simulink model "Therealone"  (R2023b)
settings: Solver=VariableStepAuto  StartTime=0.0  StopTime=1  RelTol=1e-3
libraries: spsSeriesRLCBranchLib x4, spsDiodeLib x3, spsMeanLib x2, spsCurrentMeasurementLib x2, spsPVArrayLib x2, spsVoltageMeasurementLib x2, spsIGBTDiodeLib x1, sps_lib x1
settings Model: Creator=PC  LastModifiedBy=PC
settings DataIOCC: ReturnWorkspaceOutputs=off

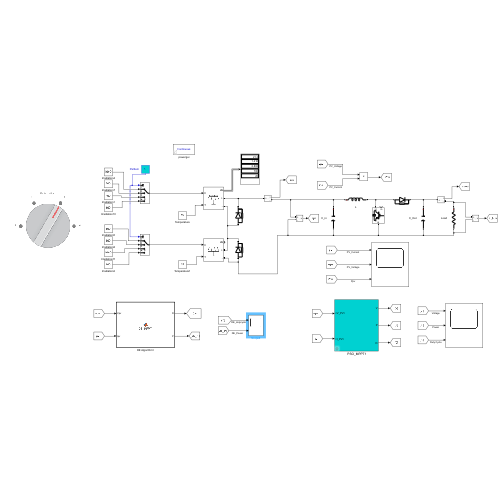
[thumbnail: Simulink's stored preview of the top-level diagram]
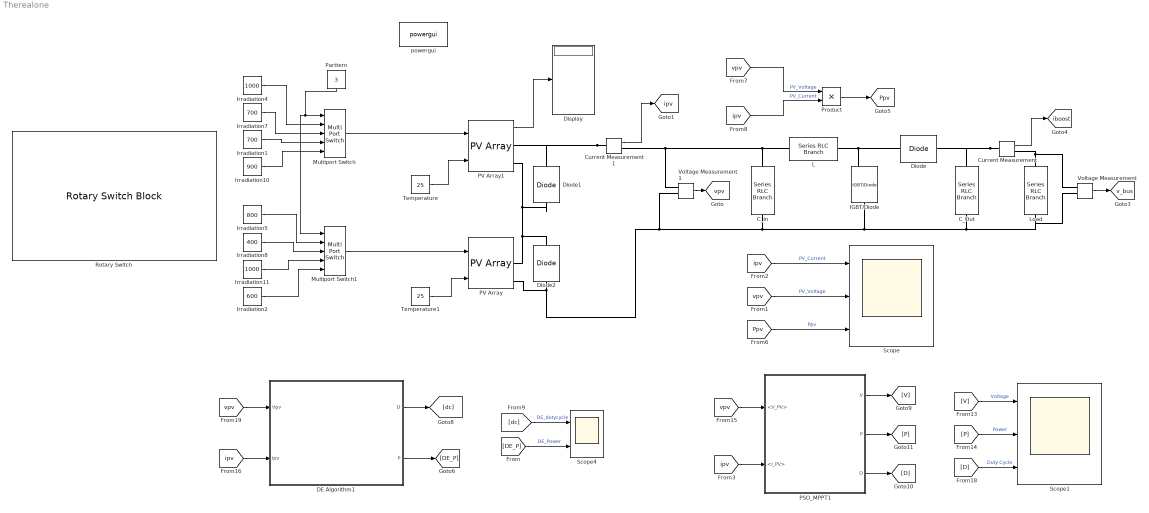
== system Therealone ==
  " PSO_MPPT1" : Subsystem  mask(MPPT PSO Block){Fsw=7812.5, n=4, w=0.1, c1=1, c2=1}
      mask prompts: Fsw "PWM Switching frequency (Hz):"; n "Number of particles (3-8)"; w "Inertia Weightage (w)"; c1 "Acceleration Coefficient (c1)"; c2 "Acceleration Coefficient (c2)"
      mask help:
      | MPPT PSO Block
      | Developed by Koh Jia Shun and Rodney Tan (PhD)
      | Version 1.00
      |
      | This block perform photovoltiac panel Maximum Power Point Tracking based on Particle Swarm Optimization algorithm.
      | This MPPT PSO method is implemented using MATLAB code scripted in MATLAB function block.
      | This MPPT PSO block take in Voltage and Current from photovoltaic panel and output PWM switching signal to drive DC converter
      mask Help:
      | <b><u>Block Setting</u></b>
      | <b>PWM Switching Frequency (Hz)</b>
      | Specify the PWM switching frequency in Hz.
      | 
      | <b>PWM Duty Cycle Step Size</b>
      | Specify the PWM duty cycle (delta) step size. Default value is 1e-5.
      mask TypeOptions Fsw:
      | PWM Generator
      | (DC-DC)/Fsw
  C_Out : spsSeriesRLCBranchLib/Series RLC Branch  LConnTagsString=__new0  RConnTagsString=__new0  BranchType=C  Resistance=1e-4  Inductance=1e-3  SetiL0=off  InitialCurrent=0  Capacitance=1*10^-3  Setx0=off  InitialVoltage=0  Measurements=None
  C_in : spsSeriesRLCBranchLib/Series RLC Branch  LConnTagsString=__new0  RConnTagsString=__new0  BranchType=C  Resistance=1e-4  Inductance=1e-3  SetiL0=off  InitialCurrent=0  Capacitance=1*10^-3  Setx0=off  InitialVoltage=0  Measurements=None
  Current Measurement : spsCurrentMeasurementLib/Current Measurement  PhasorSimulation=off  OutputType=Complex  PSBequivalent=0
  Current Measurement1 : spsCurrentMeasurementLib/Current Measurement  PhasorSimulation=off  OutputType=Complex  PSBequivalent=0
  DE Algorithm1 : MATLAB Function  TreatAsAtomicUnit=on
  Diode : spsDiodeLib/Diode  Ron=0.001  Lon=0  Vf=0.6  IC=0  UseSnubber=0  Rs=500  Cs=250e-9  Measurements=off
  Diode1 : spsDiodeLib/Diode  Ron=0.001  Lon=0  Vf=0.6  IC=0  UseSnubber=0  Rs=500  Cs=250e-9  Measurements=off
  Diode2 : spsDiodeLib/Diode  Ron=0.001  Lon=0  Vf=0.6  IC=0  UseSnubber=0  Rs=500  Cs=250e-9  Measurements=off
  Display : Display
  IGBT/Diode : spsIGBTDiodeLib/IGBT//Diode  Ron=3  Rs=1e5  Cs=inf  Measurements=off
  Irradiation1 : Constant  Value=700
  Irradiation10 : Constant  Value=900
  Irradiation11 : Constant  Value=1000
  Irradiation2 : Constant  Value=600
  Irradiation4 : Constant  Value=1000
  Irradiation5 : Constant  Value=800
  Irradiation7 : Constant  Value=700
  Irradiation8 : Constant  Value=400
  L : spsSeriesRLCBranchLib/Series RLC Branch  LConnTagsString=__new0  RConnTagsString=__new0  BranchType=L  Resistance=0.1  Inductance=3.35*10^-4  SetiL0=off  InitialCurrent=0  Capacitance=100e-6  Setx0=off  InitialVoltage=0  Measurements=None
  Load : spsSeriesRLCBranchLib/Series RLC Branch  LConnTagsString=__new0  RConnTagsString=__new0  BranchType=R  Resistance=30  Inductance=1e-3  SetiL0=off  InitialCurrent=0  Capacitance=3300e-6  Setx0=off  InitialVoltage=0  Measurements=None
  Multiport Switch : MultiPortSwitch  Inputs=4  SaturateOnIntegerOverflow=off  InputSameDT=off
  Multiport Switch1 : MultiPortSwitch  Inputs=4  SaturateOnIntegerOverflow=off  InputSameDT=off
  PV Array : spsPVArrayLib/PV Array  Npar=1  Nser=1  PlotType=array @ 25 deg.C & specified irradiances  S_vec="[ 1000  900  800 700 600 ]"  Temp_C_vec="[ 45 25  ]"  ModuleName=User-defined  PlotWhenSelected=off  Pm=100.144  Ncell=36  Voc=22.6  Isc=6.09  Vm=17.6  Im=5.69  beta_Voc_pc=-0.36099  alpha_Isc_pc=0.102  beta_Voc=-0.081584  alpha_Isc=0.0062118  IL=6.106  I0=2.2721e-10  nI=1.0181  Rsh=272.7973  Rs=0.40643  RobustModel=off  RobustCellTemperature=313.3991  BAL=on  Tc=1e-6  Tfilter=5e-5
  PV Array1 : spsPVArrayLib/PV Array  Npar=1  Nser=1  PlotType=array @ 25 deg.C & specified irradiances  S_vec="[ 1000  900  800 700 600 ]"  Temp_C_vec="[ 45 25  ]"  ModuleName=User-defined  PlotWhenSelected=off  Pm=100.144  Ncell=36  Voc=22.6  Isc=6.09  Vm=17.6  Im=5.69  beta_Voc_pc=-0.36099  alpha_Isc_pc=0.102  beta_Voc=-0.081584  alpha_Isc=0.0062118  IL=6.106  I0=2.2721e-10  nI=1.0181  Rsh=272.7973  Rs=0.40643  RobustModel=off  RobustCellTemperature=313.3991  BAL=on  Tc=1e-6  Tfilter=5e-5
  "Parttern " : Constant  Value=3
  Product : Product
  Rotary Switch : RotarySwitchBlock
      settings: Values={{'1', '2', '3', '4'}, [1 2 3 4]}
  Scope : Scope  NumInputPorts=3
  Scope1 : Scope  NumInputPorts=3
  Scope4 : Scope  NumInputPorts=2
  Temperature : Constant  Value=25
  Temperature1 : Constant  Value=25
  Voltage Measurement : spsVoltageMeasurementLib/Voltage Measurement  PhasorSimulation=off  OutputType=Complex  PSBequivalent=0
  Voltage Measurement1 : spsVoltageMeasurementLib/Voltage Measurement  PhasorSimulation=off  OutputType=Complex  PSBequivalent=0
  powergui : sps_lib/powergui  Priority=1  SimulationMode=Continuous  SampleTime=50e-6  frequency=60  Iterations=50  frequencyindice=0  Pbase=100e6  ErrMax=1e-4  UnitsV=kV  UnitsW=MW  buscounter=0  FunctionMessages=off  echomessages=off  EnableUseOfTLC=off  CurrentSourceSwitches=off  DisableSnubberDevices=off  DisableRonSwitches=off  DisableVfSwitches=off  DisplayEquations=off  AutomaticDiscreteSolvers=off  SolverType=Tustin/Backward Euler (TBE)  Interpol=off  ExternalGateDelay=off  methode=off  Ts=100  x0status=blocks  SPID=on  SwTol=0  HookPort=off  NonlinearTolerance=1e-4  nMaxIteration=100  ContinueOnMaxIteration=off  RestoreLinks=warning  ResistiveCurrentMeasurement=off  Frange=[0:2:500]  Ylog=off  Xlog=on  ShowGrid=off  save=off  variable=ZData  structure=0  ZoomFFT=off  StartTime=0.0  cycles=1  DisplayStyle=1  fundamental=60  FreqAxis=off  MaxFrequency=1000  frequencyindicesteady=1  RmsSteady=1  display=off
  tag scope: Ppv=global, iboost=global, ipv=global, v_bus=global, vpv=global
  wires:
  [ipv] -> Product/2  "PV_Current"
  Irradiation11/1 -> Multiport Switch1/4
  Irradiation8/1 -> Multiport Switch1/3
  Irradiation4/1 -> Multiport Switch/2
  Voltage Measurement1/1 -> [vpv]
  Voltage Measurement/1 -> [v_bus]
  Irradiation10/1 -> Multiport Switch/5
  Current Measurement/1 -> [iboost]
  Temperature/1 -> PV Array1/2
  Irradiation7/1 -> Multiport Switch/3
  Irradiation5/1 -> Multiport Switch1/2
  Current Measurement1/1 -> [ipv]
  Product/1 -> [Ppv]
  [vpv] -> Product/1  "PV_Voltage"
  "Parttern "/1 -> Multiport Switch1/1, Multiport Switch/1
  Temperature1/1 -> PV Array/2
  Irradiation1/1 -> Multiport Switch/4
  Irradiation2/1 -> Multiport Switch1/5
  [Ppv] -> Scope/3  "Ppv"
  [vpv] -> Scope/2  "PV_Voltage"
  [ipv] -> Scope/1  "PV_Current"
  PV Array1/1 -> Display/1
  Multiport Switch/1 -> PV Array1/1
  Multiport Switch1/1 -> PV Array/1
  [D] -> Scope1/3  "Duty Cycle"
  [V] -> Scope1/1  "Voltage"
  " PSO_MPPT1"/2(P) -> [P]
  [ipv] -> " PSO_MPPT1"/2(<I_PV>)
  [P] -> Scope1/2  "Power"
  " PSO_MPPT1"/3(D) -> [D]
  [vpv] -> " PSO_MPPT1"/1(<V_PV>)
  " PSO_MPPT1"/1(V) -> [V]
  [ipv] -> DE Algorithm1/2(Ipv)
  [dc] -> Scope4/1  "DE_dutycycle"
  [vpv] -> DE Algorithm1/1(Vpv)
  DE Algorithm1/1(D) -> [dc]
  DE Algorithm1/2(P) -> [DE_P]
  [DE_P] -> Scope4/2  "DE_Power"
  connections:
  Current Measurement1/LConn1 -- PV Array1/RConn1 -- Diode1/RConn1
  Diode2/LConn1 -- C_in/RConn1 -- Voltage Measurement/LConn2 -- Load/RConn1 -- C_Out/RConn1 -- IGBT/Diode/RConn1 -- Voltage Measurement1/LConn2 -- PV Array/RConn2
  Voltage Measurement1/LConn1 -- Current Measurement1/RConn1 -- C_in/LConn1 -- L/LConn1
  Diode1/LConn1 -- PV Array1/RConn2 -- PV Array/RConn1 -- Diode2/RConn1
  Voltage Measurement/LConn1 -- Current Measurement/RConn1 -- Load/LConn1
  Current Measurement/LConn1 -- Diode/RConn1 -- C_Out/LConn1
  L/RConn1 -- Diode/LConn1 -- IGBT/Diode/LConn1

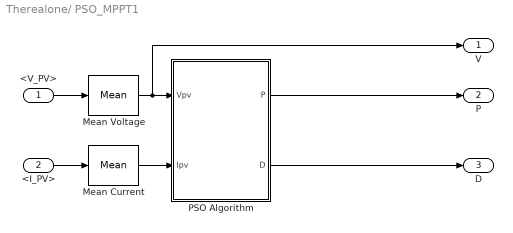
== system Therealone/ PSO_MPPT1 ==
  <V_PV> : Inport
  <I_PV> : Inport  Port=2
  Mean Current : spsMeanLib/Mean  Freq=Fsw  Vinit=0  Ts=0
  Mean Voltage : spsMeanLib/Mean  Freq=Fsw  Vinit=0  Ts=0
  PSO Algorithm : MATLAB Function  TreatAsAtomicUnit=on
  V : Outport  VectorParamsAs1DForOutWhenUnconnected=off
  P : Outport  Port=2  VectorParamsAs1DForOutWhenUnconnected=off
  D : Outport  Port=3  VectorParamsAs1DForOutWhenUnconnected=off
  wires:
  Mean Voltage/1 -> PSO Algorithm/1(Vpv), V/1
  Mean Current/1 -> PSO Algorithm/2(Ipv)
  PSO Algorithm/1(P) -> P/1
  PSO Algorithm/2(D) -> D/1
  <V_PV>/1 -> Mean Voltage/1
  <I_PV>/1 -> Mean Current/1

== matlab function Therealone/ PSO_MPPT1/PSO Algorithm ==
  settings: updateMethod=DISCRETE  sampleTime=0.002
  data: P output; Vpv input; D output; n parameter; w parameter; c1 parameter; c2 parameter; Ipv input
function [P,D]= PSO(Vpv, n, w, c1, c2, Ipv)
    %Initialisation
    % u = current particle, dcurrent= current duty cycle, pbest= best duty cycle
    % p = power of positions, dc = duty cycle of positions, v=velocity(delta duty cycle)
    % counter = time for transient, gbest = best duty cycle
    
    coder.extrinsic('randi')
    P=Vpv*Ipv;

    persistent idx u dcurrent pbest p dc v gbest n_particle Pprev k bool  closeness r;
    
    if(isempty(p))
        bool =0;
        k=0;
        idx=0;
        closeness = false;
        Pprev=Vpv*Ipv;
        n_particle=n;
        dcurrent=0.5;
        gbest=0.5;
        p=zeros(n_particle,1);
        r=zeros(2,1);
        v=zeros(n_particle,1);
        pbest=zeros(n_particle,1);
        u=0;
        dc=zeros(n_particle,1);

        
        if(n_particle ==3)
            dc(1)=randi( [5 330])/1000;
            dc(2)=randi( [330 660])/1000;
            dc(3)=randi( [660 995])/1000;
            
        end 
        if(n_particle ==4)
            dc(1)=randi( [5 250])/1000;
            dc(2)=randi( [250 500])/1000;
            dc(3)=randi( [500 750])/1000;
            dc(4)=randi( [760 995])/1000;
        end 
        
        if(n_particle ==5)
            dc(1)=randi( [5 200])/1000;
            dc(2)=randi( [200 400])/1000;
            dc(3)=randi( [400 600])/1000;
            dc(4)=randi( [600 800])/1000;
            dc(5)=randi( [800 995])/1000;

        end 
        if(n_particle ==6)
            dc(1)=randi( [5 166])/1000;
            dc(2)=randi( [166 333])/1000;
            dc(3)=randi( [333 500])/1000;
            dc(4)=randi( [500 666])/1000;
            dc(5)=randi( [666 833])/1000;
            dc(6)=randi( [833 995])/1000;
        end 
        if(n_particle ==7)
            dc(1)=randi( [5 143])/1000;
            dc(2)=randi( [143 286])/1000;
            dc(3)=randi( [286 429])/1000;
            dc(4)=randi( [429 571])/1000;
            dc(5)=randi( [571 714])/1000;
            dc(6)=randi( [714 857])/1000;
            dc(7)=randi( [857 995])/1000;
        end 
        if(n_particle ==8)
            dc(1)=randi( [5 100])/1000;
            dc(2)=randi( [150 250])/1000;
            dc(3)=randi( [250 350])/1000;
            dc(4)=randi( [350 500])/1000;
            dc(5)=randi( [500 650])/1000;
            dc(6)=randi( [650 750])/1000;
            dc(7)=randi( [750 850])/1000;
            dc(8)=randi( [900 1000])/1000;
        end 
    end
    
    D=dcurrent;


    %after counter end counting, power is stable after transient.
    %if power is larger than current power, current best position is updated
    %with new power

    if(u>=1 && u<=n_particle)
        if((Vpv*Ipv)>p(u))
            p(u)=Vpv*Ipv;
            pbest(u)=dcurrent;
        end
    end
    u=u+1;
    
    %when gbest is updated, when u+1 again, it will reset to u=1,2,3... to
    %update duty cycle again

    if(u > n_particle+1)
        u=1;
    end

    if(u == n_particle+1 )   %eg if number of particle =4 after all 4 particle is tested with new position(duty cycle)and get fitness value(power)
        
        if(bool==0)
            k=k+1;    
        end
        
        
        [~,idx]=max(p);
        gbest=pbest(idx);      % at 5th iteration(update gbest) and velocity(delta duty cycle) of all particles
        if(bool ==0)
            D=gbest;
        else
            D=dc(idx); %mean
        end
        dcurrent=D;
        %update velocity and duty cycle
        if(bool==0)
            for j=1:n_particle
                r(1)= randi( [1 30])/100;
                r(2) = randi( [5 30])/100;
                v(j)=updatevelocity(w,c1,c2,v(j),pbest(j),dc(j),gbest);
                dc(j)=updateduty(dc(j),v(j));
            end
        end
        %wait for stable after reinitialization
        
        
        if(bool==0)
            closeness=true;
            for i=1:n_particle
               for j=1:n_particle
                if(i~=j)
                   closeness = closeness &  (abs(dc(i)-dc(j))<0.1); % 0.05
                end
               end
            end
        end
        
        %if the power stables already
        if(bool==1 )
            
            %check if the power changes
            if(abs(Vpv*Ipv-Pprev)/Pprev >= 0.05)%0.1
                idx=0;
                dcurrent=0.5;
                gbest=0.5;
                p=zeros(n_particle,1);
                v=zeros(n_particle,1);
                pbest=zeros(n_particle,1);
                dc=zeros(n_particle,1);
                if(n_particle ==3)
                    dc(1)=randi( [5 330])/1000;
                    dc(2)=randi( [330 660])/1000;
                    dc(3)=randi( [660 995])/1000;

                end 
                if(n_particle ==4)
                    dc(1)=randi( [5 250])/1000;
                    dc(2)=randi( [250 500])/1000;
                    dc(3)=randi( [500 750])/1000;
                    dc(4)=randi( [760 995])/1000;
                end 

                if(n_particle ==5)
                    dc(1)=randi( [5 200])/1000;
                    dc(2)=randi( [200 400])/1000;
                    dc(3)=randi( [400 600])/1000;
                    dc(4)=randi( [600 800])/1000;
                    dc(5)=randi( [800 995])/1000;

                end 
                if(n_particle ==6)
                    dc(1)=randi( [5 166])/1000;
                    dc(2)=randi( [166 333])/1000;
                    dc(3)=randi( [333 500])/1000;
                    dc(4)=randi( [500 666])/1000;
                    dc(5)=randi( [666 833])/1000;
                    dc(6)=randi( [833 995])/1000;
                end 
                if(n_particle ==7)
                    dc(1)=randi( [5 143])/1000;
                    dc(2)=randi( [143 286])/1000;
                    dc(3)=randi( [286 429])/1000;
                    dc(4)=randi( [429 571])/1000;
                    dc(5)=randi( [571 714])/1000;
                    dc(6)=randi( [714 857])/1000;
                    dc(7)=randi( [857 995])/1000;
                end 
                if(n_particle ==8)
                    dc(1)=randi( [5 100])/1000;
                    dc(2)=randi( [150 250])/1000;
                    dc(3)=randi( [250 350])/1000;
                    dc(4)=randi( [350 500])/1000;
                    dc(5)=randi( [500 650])/1000;
                    dc(6)=randi( [650 750])/1000;
                    dc(7)=randi( [750 850])/1000;
                    dc(8)=randi( [900 1000])/1000;
                end
                
                bool=0;
            
            end
      
        end
        
        if(closeness==1)
            bool=1; 
            closeness=false;   
        end
    
        if(k>70)
                idx=0;
                dcurrent=0.5;
                gbest=0.5;
                p=zeros(n_particle,1);
                v=zeros(n_particle,1);
                pbest=zeros(n_particle,1);
                dc=zeros(n_particle,1);
                
                
                if(n_particle ==3)
                    dc(1)=randi( [5 330])/1000;
                    dc(2)=randi( [330 660])/1000;
                    dc(3)=randi( [660 995])/1000;

                end 
                if(n_particle ==4)
                    dc(1)=randi( [5 250])/1000;
                    dc(2)=randi( [250 500])/1000;
                    dc(3)=randi( [500 750])/1000;
                    dc(4)=randi( [760 995])/1000;
                end 

                if(n_particle ==5)
                    dc(1)=randi( [5 200])/1000;
                    dc(2)=randi( [200 400])/1000;
                    dc(3)=randi( [400 600])/1000;
                    dc(4)=randi( [600 800])/1000;
                    dc(5)=randi( [800 995])/1000;

                end 
                if(n_particle ==6)
                    dc(1)=randi( [5 166])/1000;
                    dc(2)=randi( [166 333])/1000;
                    dc(3)=randi( [333 500])/1000;
                    dc(4)=randi( [500 666])/1000;
                    dc(5)=randi( [666 833])/1000;
                    dc(6)=randi( [833 995])/1000;
                end 
                if(n_particle ==7)
                    dc(1)=randi( [5 143])/1000;
                    dc(2)=randi( [143 286])/1000;
                    dc(3)=randi( [286 429])/1000;
                    dc(4)=randi( [429 571])/1000;
                    dc(5)=randi( [571 714])/1000;
                    dc(6)=randi( [714 857])/1000;
                    dc(7)=randi( [857 995])/1000;
                end 
                if(n_particle ==8)
                    dc(1)=randi( [5 100])/1000;
                    dc(2)=randi( [150 250])/1000;
                    dc(3)=randi( [250 350])/1000;
                    dc(4)=randi( [350 500])/1000;
                    dc(5)=randi( [500 650])/1000;
                    dc(6)=randi( [650 750])/1000;
                    dc(7)=randi( [750 850])/1000;
                    dc(8)=randi( [900 1000])/1000;
                end
                k=0;
        end
        
        Pprev = Vpv*Ipv;
        
        
        return;
    else
        %update each particle's duty cycle, reset counter. 
        if(bool==0)
            D=dc(u);
        else
            D=dc(idx); %mean 
          
        end
        dcurrent=D;
        return; 
    end
    
end

function vfinal=updatevelocity(w,c1,c2,velocity,pobest,d,gwbest)
    % PSO Parameters
    vfinal = (w*velocity)+(c1*rand(1)*(pobest-d))+(c2*rand(1)*(gwbest-d));
    
    
end

function dfinal=updateduty(d,velocity)

    dup=d+velocity;
    if(dup>1)
        dfinal=1;
    elseif(dup<0)
        dfinal=0;
    else
        dfinal=dup;
    end
end

== matlab function Therealone/DE Algorithm1 ==
  settings: updateMethod=DISCRETE
  data: D output; Vpv input; Ipv input; P output
function [D,P] = DE_MPPT(Vpv, Ipv)
    n = 3;
    
    % Differential Evolution Parameters
    F = 0.5;    % Differential weight
    CR = 0.9;   % Crossover rate
    
    % Initialization
    coder.extrinsic('randi');
    P = Vpv * Ipv;
    
    persistent population fitness best_individual n_particle;
    
    % Initialize persistent variables
    if(isempty(population))
        n_particle = n;
        population = rand(n_particle, 1);  % Initialize with random values between 0 and 1
        fitness = zeros(n_particle, 1);
        best_individual = rand();  % Initialize with a random value between 0 and 1
    end
    
    % Evaluate fitness of each individual in the population
    for i = 1:n_particle
        fitness(i) = objective_function(population(i), Vpv, Ipv);
        
        % Update the best individual
        if fitness(i) > objective_function(best_individual, Vpv, Ipv)
            best_individual = population(i);
        end
    end
    
    % Update the population using Differential Evolution
    for i = 1:n_particle
        % Select three distinct individuals different from the current one
        candidates = randperm(n_particle, 3);
        a = candidates(1);
        b = candidates(2);
        c = candidates(3);
        
        % Generate a trial vector using DE mutation and crossover
        trial_vector = population(a) + F * (population(b) - population(c));
        if rand() <= CR
            % Perform crossover
            population(i) = trial_vector;
        end
    end
    
    % Select the best individual from the current population
    [~, idx] = max(fitness);
    D = population(idx);
    
    % Objective function to maximize (you can replace this with your own)
    function value = objective_function(x, Vpv, Ipv)
        % Replace this with your own objective function to be optimized
        P = (Vpv * Ipv)+ x;  % Example: Power is proportional to the duty cycle
        value = P;
    end
end
